simulink model "gm_hybrid_lht"  (R2019b)
settings: Solver=FixedStepDiscrete  StartTime=0.0  StopTime=inf  FixedStep=1/120e6  RelTol=1e-3
undefined symbols (not defined in the file or in its folder): bt, height, nTheta, width
libraries: hdlsllib x312, simulink x194, hdlmdlgenlib x7, dspsrcs4 x1
(part 6 of 13)

== system gm_hybrid_lht/Hybrid LHT/Hybrid LHT Accumulator/Accumulator with Switches/Accumulator_instance56 ==
  shift : Inport  OutDataTypeStr=fixdt(0, 6, 0)  PortDimensions=1  SampleTime=8.33333333333333e-09
  mode : Inport  Port=2  OutDataTypeStr=boolean  PortDimensions=1  SampleTime=8.33333333333333e-09
  address : Inport  Port=3  OutDataTypeStr=fixdt(0, 10, 0)  PortDimensions=1  SampleTime=8.33333333333333e-09
  edge : Inport  Port=4  OutDataTypeStr=boolean  PortDimensions=1  SampleTime=8.33333333333333e-09
  AND : Logic  IconShape=distinctive  AllPortsSameDT=off  OutDataTypeStr=boolean
  Add : Sum  OutDataTypeStr=fixdt(0, ceil(log2(maxRho*2)), 0)
  Bit Concat : hdlsllib/Logic and Bit Operations/Bit Concat  numInputs=2
      settings: SourceProductName=Simulink
  Bit Slice : hdlsllib/Logic and Bit Operations/Bit Slice  lidx=voteWL-1  ridx=0
  Bitwise AND : simulink/Logic and Bit Operations/Bitwise Operator  logicop=AND  UseBitMask=off  NumInputPorts=2  BitMask=bin2dec('11011001')  BitMaskRealWorld=Stored Integer
  Bitwise NOT : simulink/Logic and Bit Operations/Bitwise Operator  logicop=NOT  UseBitMask=off  BitMask=bin2dec('11011001')  BitMaskRealWorld=Stored Integer
  Bitwise OR : simulink/Logic and Bit Operations/Bitwise Operator  logicop=OR  UseBitMask=off  NumInputPorts=2  BitMask=bin2dec('11011001')  BitMaskRealWorld=Stored Integer
  Block RAM : Subsystem
  Constant : Constant  Value=0  OutDataTypeStr=fixdt(0, 36-voteWL, 0)  SampleTime=-1
  Constant1 : Constant  Value=2^(voteWL)-1  OutDataTypeStr=fixdt(0, 36, 0)  SampleTime=-1
  Delay{,1..2,4..5} (5 alike) : Delay  DelayLength=1
  Multiport Switch : MultiPortSwitch  DataPortOrder=Zero-based contiguous  Inputs=2  zeroidx=on
  Multiport Switch1 : MultiPortSwitch  DataPortOrder=Zero-based contiguous  Inputs=2  zeroidx=on
  Relational Operator : RelationalOperator  Operator===  OutDataTypeStr=boolean  RndMeth=Simplest
  Shift Arithmetic : ArithShift  BitShiftNumberSource=Input port  BitShiftNumber=8  BitShiftDirection=Left  DiagnosticForOORShift=Error
      settings: InputPortMap=u0,p1
  Shift Arithmetic1 : ArithShift  BitShiftNumberSource=Input port  BitShiftNumber=8  BitShiftDirection=Left  DiagnosticForOORShift=Error
      settings: InputPortMap=u0,p1
  Shift Arithmetic2 : ArithShift  BitShiftNumberSource=Input port  BitShiftNumber=8  BitShiftDirection=Right  DiagnosticForOORShift=Error
      settings: InputPortMap=u0,p1
  Signal Specification : SignalSpecification  OutDataTypeStr=fixdt(0, 36, 0)
  Vote : Constant  OutDataTypeStr=fixdt(0,1,0)  SampleTime=-1
  Zero : Constant  Value=0  OutDataTypeStr=fixdt(0,1,0)  SampleTime=-1
  hps : Outport
  wires:
  Block RAM/1(rd_data) -> Signal Specification/1
  Multiport Switch1/1 -> Shift Arithmetic2/1, Bitwise AND/2
  Signal Specification/1 -> Multiport Switch1/2
  Bitwise OR/1 -> Block RAM/1(wr_data), Delay5/1
  Bitwise AND/1 -> Bitwise OR/1
  Shift Arithmetic2/1 -> Bit Slice/1
  Add/1 -> Multiport Switch/3
  Multiport Switch/1 -> Bit Concat/2
  Bit Concat/1 -> Shift Arithmetic/1
  Shift Arithmetic/1 -> Bitwise OR/2
  Delay5/1 -> Multiport Switch1/3
  edge/1 -> Delay1/1
  address/1 -> Block RAM/4(rd_addr), Delay/1, Relational Operator/2
  mode/1 -> Multiport Switch/1
  shift/1 -> Delay4/1
  AND/1 -> Delay2/1
  Bit Slice/1 -> Add/2, hps/1
  Bitwise NOT/1 -> Bitwise AND/1
  Constant/1 -> Bit Concat/1
  Constant1/1 -> Shift Arithmetic1/1
  Delay/1 -> Block RAM/2(wr_addr), Relational Operator/1
  Delay1/1 -> Block RAM/3(wr_en), AND/1
  Delay2/1 -> Multiport Switch1/1
  Delay4/1 -> Shift Arithmetic2/2, Shift Arithmetic/2, Shift Arithmetic1/2
  Relational Operator/1 -> AND/2
  Shift Arithmetic1/1 -> Bitwise NOT/1
  Vote/1 -> Add/1
  Zero/1 -> Multiport Switch/2

== system gm_hybrid_lht/Hybrid LHT/Hybrid LHT Accumulator/Accumulator with Switches/Accumulator_instance57 ==
  shift : Inport  OutDataTypeStr=fixdt(0, 6, 0)  PortDimensions=1  SampleTime=8.33333333333333e-09
  mode : Inport  Port=2  OutDataTypeStr=boolean  PortDimensions=1  SampleTime=8.33333333333333e-09
  address : Inport  Port=3  OutDataTypeStr=fixdt(0, 10, 0)  PortDimensions=1  SampleTime=8.33333333333333e-09
  edge : Inport  Port=4  OutDataTypeStr=boolean  PortDimensions=1  SampleTime=8.33333333333333e-09
  AND : Logic  IconShape=distinctive  AllPortsSameDT=off  OutDataTypeStr=boolean
  Add : Sum  OutDataTypeStr=fixdt(0, ceil(log2(maxRho*2)), 0)
  Bit Concat : hdlsllib/Logic and Bit Operations/Bit Concat  numInputs=2
      settings: SourceProductName=Simulink
  Bit Slice : hdlsllib/Logic and Bit Operations/Bit Slice  lidx=voteWL-1  ridx=0
  Bitwise AND : simulink/Logic and Bit Operations/Bitwise Operator  logicop=AND  UseBitMask=off  NumInputPorts=2  BitMask=bin2dec('11011001')  BitMaskRealWorld=Stored Integer
  Bitwise NOT : simulink/Logic and Bit Operations/Bitwise Operator  logicop=NOT  UseBitMask=off  BitMask=bin2dec('11011001')  BitMaskRealWorld=Stored Integer
  Bitwise OR : simulink/Logic and Bit Operations/Bitwise Operator  logicop=OR  UseBitMask=off  NumInputPorts=2  BitMask=bin2dec('11011001')  BitMaskRealWorld=Stored Integer
  Block RAM : Subsystem
  Constant : Constant  Value=0  OutDataTypeStr=fixdt(0, 36-voteWL, 0)  SampleTime=-1
  Constant1 : Constant  Value=2^(voteWL)-1  OutDataTypeStr=fixdt(0, 36, 0)  SampleTime=-1
  Delay{,1..2,4..5} (5 alike) : Delay  DelayLength=1
  Multiport Switch : MultiPortSwitch  DataPortOrder=Zero-based contiguous  Inputs=2  zeroidx=on
  Multiport Switch1 : MultiPortSwitch  DataPortOrder=Zero-based contiguous  Inputs=2  zeroidx=on
  Relational Operator : RelationalOperator  Operator===  OutDataTypeStr=boolean  RndMeth=Simplest
  Shift Arithmetic : ArithShift  BitShiftNumberSource=Input port  BitShiftNumber=8  BitShiftDirection=Left  DiagnosticForOORShift=Error
      settings: InputPortMap=u0,p1
  Shift Arithmetic1 : ArithShift  BitShiftNumberSource=Input port  BitShiftNumber=8  BitShiftDirection=Left  DiagnosticForOORShift=Error
      settings: InputPortMap=u0,p1
  Shift Arithmetic2 : ArithShift  BitShiftNumberSource=Input port  BitShiftNumber=8  BitShiftDirection=Right  DiagnosticForOORShift=Error
      settings: InputPortMap=u0,p1
  Signal Specification : SignalSpecification  OutDataTypeStr=fixdt(0, 36, 0)
  Vote : Constant  OutDataTypeStr=fixdt(0,1,0)  SampleTime=-1
  Zero : Constant  Value=0  OutDataTypeStr=fixdt(0,1,0)  SampleTime=-1
  hps : Outport
  wires:
  Block RAM/1(rd_data) -> Signal Specification/1
  Multiport Switch1/1 -> Shift Arithmetic2/1, Bitwise AND/2
  Signal Specification/1 -> Multiport Switch1/2
  Bitwise OR/1 -> Block RAM/1(wr_data), Delay5/1
  Bitwise AND/1 -> Bitwise OR/1
  Shift Arithmetic2/1 -> Bit Slice/1
  Add/1 -> Multiport Switch/3
  Multiport Switch/1 -> Bit Concat/2
  Bit Concat/1 -> Shift Arithmetic/1
  Shift Arithmetic/1 -> Bitwise OR/2
  Delay5/1 -> Multiport Switch1/3
  edge/1 -> Delay1/1
  address/1 -> Block RAM/4(rd_addr), Delay/1, Relational Operator/2
  mode/1 -> Multiport Switch/1
  shift/1 -> Delay4/1
  AND/1 -> Delay2/1
  Bit Slice/1 -> Add/2, hps/1
  Bitwise NOT/1 -> Bitwise AND/1
  Constant/1 -> Bit Concat/1
  Constant1/1 -> Shift Arithmetic1/1
  Delay/1 -> Block RAM/2(wr_addr), Relational Operator/1
  Delay1/1 -> Block RAM/3(wr_en), AND/1
  Delay2/1 -> Multiport Switch1/1
  Delay4/1 -> Shift Arithmetic2/2, Shift Arithmetic/2, Shift Arithmetic1/2
  Relational Operator/1 -> AND/2
  Shift Arithmetic1/1 -> Bitwise NOT/1
  Vote/1 -> Add/1
  Zero/1 -> Multiport Switch/2

== system gm_hybrid_lht/Hybrid LHT/Hybrid LHT Accumulator/Accumulator with Switches/Accumulator_instance58 ==
  shift : Inport  OutDataTypeStr=fixdt(0, 6, 0)  PortDimensions=1  SampleTime=8.33333333333333e-09
  mode : Inport  Port=2  OutDataTypeStr=boolean  PortDimensions=1  SampleTime=8.33333333333333e-09
  address : Inport  Port=3  OutDataTypeStr=fixdt(0, 10, 0)  PortDimensions=1  SampleTime=8.33333333333333e-09
  edge : Inport  Port=4  OutDataTypeStr=boolean  PortDimensions=1  SampleTime=8.33333333333333e-09
  AND : Logic  IconShape=distinctive  AllPortsSameDT=off  OutDataTypeStr=boolean
  Add : Sum  OutDataTypeStr=fixdt(0, ceil(log2(maxRho*2)), 0)
  Bit Concat : hdlsllib/Logic and Bit Operations/Bit Concat  numInputs=2
      settings: SourceProductName=Simulink
  Bit Slice : hdlsllib/Logic and Bit Operations/Bit Slice  lidx=voteWL-1  ridx=0
  Bitwise AND : simulink/Logic and Bit Operations/Bitwise Operator  logicop=AND  UseBitMask=off  NumInputPorts=2  BitMask=bin2dec('11011001')  BitMaskRealWorld=Stored Integer
  Bitwise NOT : simulink/Logic and Bit Operations/Bitwise Operator  logicop=NOT  UseBitMask=off  BitMask=bin2dec('11011001')  BitMaskRealWorld=Stored Integer
  Bitwise OR : simulink/Logic and Bit Operations/Bitwise Operator  logicop=OR  UseBitMask=off  NumInputPorts=2  BitMask=bin2dec('11011001')  BitMaskRealWorld=Stored Integer
  Block RAM : Subsystem
  Constant : Constant  Value=0  OutDataTypeStr=fixdt(0, 36-voteWL, 0)  SampleTime=-1
  Constant1 : Constant  Value=2^(voteWL)-1  OutDataTypeStr=fixdt(0, 36, 0)  SampleTime=-1
  Delay{,1..2,4..5} (5 alike) : Delay  DelayLength=1
  Multiport Switch : MultiPortSwitch  DataPortOrder=Zero-based contiguous  Inputs=2  zeroidx=on
  Multiport Switch1 : MultiPortSwitch  DataPortOrder=Zero-based contiguous  Inputs=2  zeroidx=on
  Relational Operator : RelationalOperator  Operator===  OutDataTypeStr=boolean  RndMeth=Simplest
  Shift Arithmetic : ArithShift  BitShiftNumberSource=Input port  BitShiftNumber=8  BitShiftDirection=Left  DiagnosticForOORShift=Error
      settings: InputPortMap=u0,p1
  Shift Arithmetic1 : ArithShift  BitShiftNumberSource=Input port  BitShiftNumber=8  BitShiftDirection=Left  DiagnosticForOORShift=Error
      settings: InputPortMap=u0,p1
  Shift Arithmetic2 : ArithShift  BitShiftNumberSource=Input port  BitShiftNumber=8  BitShiftDirection=Right  DiagnosticForOORShift=Error
      settings: InputPortMap=u0,p1
  Signal Specification : SignalSpecification  OutDataTypeStr=fixdt(0, 36, 0)
  Vote : Constant  OutDataTypeStr=fixdt(0,1,0)  SampleTime=-1
  Zero : Constant  Value=0  OutDataTypeStr=fixdt(0,1,0)  SampleTime=-1
  hps : Outport
  wires:
  Block RAM/1(rd_data) -> Signal Specification/1
  Multiport Switch1/1 -> Shift Arithmetic2/1, Bitwise AND/2
  Signal Specification/1 -> Multiport Switch1/2
  Bitwise OR/1 -> Block RAM/1(wr_data), Delay5/1
  Bitwise AND/1 -> Bitwise OR/1
  Shift Arithmetic2/1 -> Bit Slice/1
  Add/1 -> Multiport Switch/3
  Multiport Switch/1 -> Bit Concat/2
  Bit Concat/1 -> Shift Arithmetic/1
  Shift Arithmetic/1 -> Bitwise OR/2
  Delay5/1 -> Multiport Switch1/3
  edge/1 -> Delay1/1
  address/1 -> Block RAM/4(rd_addr), Delay/1, Relational Operator/2
  mode/1 -> Multiport Switch/1
  shift/1 -> Delay4/1
  AND/1 -> Delay2/1
  Bit Slice/1 -> Add/2, hps/1
  Bitwise NOT/1 -> Bitwise AND/1
  Constant/1 -> Bit Concat/1
  Constant1/1 -> Shift Arithmetic1/1
  Delay/1 -> Block RAM/2(wr_addr), Relational Operator/1
  Delay1/1 -> Block RAM/3(wr_en), AND/1
  Delay2/1 -> Multiport Switch1/1
  Delay4/1 -> Shift Arithmetic2/2, Shift Arithmetic/2, Shift Arithmetic1/2
  Relational Operator/1 -> AND/2
  Shift Arithmetic1/1 -> Bitwise NOT/1
  Vote/1 -> Add/1
  Zero/1 -> Multiport Switch/2

== system gm_hybrid_lht/Hybrid LHT/Hybrid LHT Accumulator/Accumulator with Switches/Accumulator_instance59 ==
  shift : Inport  OutDataTypeStr=fixdt(0, 6, 0)  PortDimensions=1  SampleTime=8.33333333333333e-09
  mode : Inport  Port=2  OutDataTypeStr=boolean  PortDimensions=1  SampleTime=8.33333333333333e-09
  address : Inport  Port=3  OutDataTypeStr=fixdt(0, 10, 0)  PortDimensions=1  SampleTime=8.33333333333333e-09
  edge : Inport  Port=4  OutDataTypeStr=boolean  PortDimensions=1  SampleTime=8.33333333333333e-09
  AND : Logic  IconShape=distinctive  AllPortsSameDT=off  OutDataTypeStr=boolean
  Add : Sum  OutDataTypeStr=fixdt(0, ceil(log2(maxRho*2)), 0)
  Bit Concat : hdlsllib/Logic and Bit Operations/Bit Concat  numInputs=2
      settings: SourceProductName=Simulink
  Bit Slice : hdlsllib/Logic and Bit Operations/Bit Slice  lidx=voteWL-1  ridx=0
  Bitwise AND : simulink/Logic and Bit Operations/Bitwise Operator  logicop=AND  UseBitMask=off  NumInputPorts=2  BitMask=bin2dec('11011001')  BitMaskRealWorld=Stored Integer
  Bitwise NOT : simulink/Logic and Bit Operations/Bitwise Operator  logicop=NOT  UseBitMask=off  BitMask=bin2dec('11011001')  BitMaskRealWorld=Stored Integer
  Bitwise OR : simulink/Logic and Bit Operations/Bitwise Operator  logicop=OR  UseBitMask=off  NumInputPorts=2  BitMask=bin2dec('11011001')  BitMaskRealWorld=Stored Integer
  Block RAM : Subsystem
  Constant : Constant  Value=0  OutDataTypeStr=fixdt(0, 36-voteWL, 0)  SampleTime=-1
  Constant1 : Constant  Value=2^(voteWL)-1  OutDataTypeStr=fixdt(0, 36, 0)  SampleTime=-1
  Delay{,1..2,4..5} (5 alike) : Delay  DelayLength=1
  Multiport Switch : MultiPortSwitch  DataPortOrder=Zero-based contiguous  Inputs=2  zeroidx=on
  Multiport Switch1 : MultiPortSwitch  DataPortOrder=Zero-based contiguous  Inputs=2  zeroidx=on
  Relational Operator : RelationalOperator  Operator===  OutDataTypeStr=boolean  RndMeth=Simplest
  Shift Arithmetic : ArithShift  BitShiftNumberSource=Input port  BitShiftNumber=8  BitShiftDirection=Left  DiagnosticForOORShift=Error
      settings: InputPortMap=u0,p1
  Shift Arithmetic1 : ArithShift  BitShiftNumberSource=Input port  BitShiftNumber=8  BitShiftDirection=Left  DiagnosticForOORShift=Error
      settings: InputPortMap=u0,p1
  Shift Arithmetic2 : ArithShift  BitShiftNumberSource=Input port  BitShiftNumber=8  BitShiftDirection=Right  DiagnosticForOORShift=Error
      settings: InputPortMap=u0,p1
  Signal Specification : SignalSpecification  OutDataTypeStr=fixdt(0, 36, 0)
  Vote : Constant  OutDataTypeStr=fixdt(0,1,0)  SampleTime=-1
  Zero : Constant  Value=0  OutDataTypeStr=fixdt(0,1,0)  SampleTime=-1
  hps : Outport
  wires:
  Block RAM/1(rd_data) -> Signal Specification/1
  Multiport Switch1/1 -> Shift Arithmetic2/1, Bitwise AND/2
  Signal Specification/1 -> Multiport Switch1/2
  Bitwise OR/1 -> Block RAM/1(wr_data), Delay5/1
  Bitwise AND/1 -> Bitwise OR/1
  Shift Arithmetic2/1 -> Bit Slice/1
  Add/1 -> Multiport Switch/3
  Multiport Switch/1 -> Bit Concat/2
  Bit Concat/1 -> Shift Arithmetic/1
  Shift Arithmetic/1 -> Bitwise OR/2
  Delay5/1 -> Multiport Switch1/3
  edge/1 -> Delay1/1
  address/1 -> Block RAM/4(rd_addr), Delay/1, Relational Operator/2
  mode/1 -> Multiport Switch/1
  shift/1 -> Delay4/1
  AND/1 -> Delay2/1
  Bit Slice/1 -> Add/2, hps/1
  Bitwise NOT/1 -> Bitwise AND/1
  Constant/1 -> Bit Concat/1
  Constant1/1 -> Shift Arithmetic1/1
  Delay/1 -> Block RAM/2(wr_addr), Relational Operator/1
  Delay1/1 -> Block RAM/3(wr_en), AND/1
  Delay2/1 -> Multiport Switch1/1
  Delay4/1 -> Shift Arithmetic2/2, Shift Arithmetic/2, Shift Arithmetic1/2
  Relational Operator/1 -> AND/2
  Shift Arithmetic1/1 -> Bitwise NOT/1
  Vote/1 -> Add/1
  Zero/1 -> Multiport Switch/2

== system gm_hybrid_lht/Hybrid LHT/Hybrid LHT Accumulator/Accumulator with Switches/Accumulator_instance6 ==
  shift : Inport  OutDataTypeStr=fixdt(0, 6, 0)  PortDimensions=1  SampleTime=8.33333333333333e-09
  mode : Inport  Port=2  OutDataTypeStr=boolean  PortDimensions=1  SampleTime=8.33333333333333e-09
  address : Inport  Port=3  OutDataTypeStr=fixdt(0, 10, 0)  PortDimensions=1  SampleTime=8.33333333333333e-09
  edge : Inport  Port=4  OutDataTypeStr=boolean  PortDimensions=1  SampleTime=8.33333333333333e-09
  AND : Logic  IconShape=distinctive  AllPortsSameDT=off  OutDataTypeStr=boolean
  Add : Sum  OutDataTypeStr=fixdt(0, ceil(log2(maxRho*2)), 0)
  Bit Concat : hdlsllib/Logic and Bit Operations/Bit Concat  numInputs=2
      settings: SourceProductName=Simulink
  Bit Slice : hdlsllib/Logic and Bit Operations/Bit Slice  lidx=voteWL-1  ridx=0
  Bitwise AND : simulink/Logic and Bit Operations/Bitwise Operator  logicop=AND  UseBitMask=off  NumInputPorts=2  BitMask=bin2dec('11011001')  BitMaskRealWorld=Stored Integer
  Bitwise NOT : simulink/Logic and Bit Operations/Bitwise Operator  logicop=NOT  UseBitMask=off  BitMask=bin2dec('11011001')  BitMaskRealWorld=Stored Integer
  Bitwise OR : simulink/Logic and Bit Operations/Bitwise Operator  logicop=OR  UseBitMask=off  NumInputPorts=2  BitMask=bin2dec('11011001')  BitMaskRealWorld=Stored Integer
  Block RAM : Subsystem
  Constant : Constant  Value=0  OutDataTypeStr=fixdt(0, 36-voteWL, 0)  SampleTime=-1
  Constant1 : Constant  Value=2^(voteWL)-1  OutDataTypeStr=fixdt(0, 36, 0)  SampleTime=-1
  Delay{,1..2,4..5} (5 alike) : Delay  DelayLength=1
  Multiport Switch : MultiPortSwitch  DataPortOrder=Zero-based contiguous  Inputs=2  zeroidx=on
  Multiport Switch1 : MultiPortSwitch  DataPortOrder=Zero-based contiguous  Inputs=2  zeroidx=on
  Relational Operator : RelationalOperator  Operator===  OutDataTypeStr=boolean  RndMeth=Simplest
  Shift Arithmetic : ArithShift  BitShiftNumberSource=Input port  BitShiftNumber=8  BitShiftDirection=Left  DiagnosticForOORShift=Error
      settings: InputPortMap=u0,p1
  Shift Arithmetic1 : ArithShift  BitShiftNumberSource=Input port  BitShiftNumber=8  BitShiftDirection=Left  DiagnosticForOORShift=Error
      settings: InputPortMap=u0,p1
  Shift Arithmetic2 : ArithShift  BitShiftNumberSource=Input port  BitShiftNumber=8  BitShiftDirection=Right  DiagnosticForOORShift=Error
      settings: InputPortMap=u0,p1
  Signal Specification : SignalSpecification  OutDataTypeStr=fixdt(0, 36, 0)
  Vote : Constant  OutDataTypeStr=fixdt(0,1,0)  SampleTime=-1
  Zero : Constant  Value=0  OutDataTypeStr=fixdt(0,1,0)  SampleTime=-1
  hps : Outport
  wires:
  Block RAM/1(rd_data) -> Signal Specification/1
  Multiport Switch1/1 -> Shift Arithmetic2/1, Bitwise AND/2
  Signal Specification/1 -> Multiport Switch1/2
  Bitwise OR/1 -> Block RAM/1(wr_data), Delay5/1
  Bitwise AND/1 -> Bitwise OR/1
  Shift Arithmetic2/1 -> Bit Slice/1
  Add/1 -> Multiport Switch/3
  Multiport Switch/1 -> Bit Concat/2
  Bit Concat/1 -> Shift Arithmetic/1
  Shift Arithmetic/1 -> Bitwise OR/2
  Delay5/1 -> Multiport Switch1/3
  edge/1 -> Delay1/1
  address/1 -> Block RAM/4(rd_addr), Delay/1, Relational Operator/2
  mode/1 -> Multiport Switch/1
  shift/1 -> Delay4/1
  AND/1 -> Delay2/1
  Bit Slice/1 -> Add/2, hps/1
  Bitwise NOT/1 -> Bitwise AND/1
  Constant/1 -> Bit Concat/1
  Constant1/1 -> Shift Arithmetic1/1
  Delay/1 -> Block RAM/2(wr_addr), Relational Operator/1
  Delay1/1 -> Block RAM/3(wr_en), AND/1
  Delay2/1 -> Multiport Switch1/1
  Delay4/1 -> Shift Arithmetic2/2, Shift Arithmetic/2, Shift Arithmetic1/2
  Relational Operator/1 -> AND/2
  Shift Arithmetic1/1 -> Bitwise NOT/1
  Vote/1 -> Add/1
  Zero/1 -> Multiport Switch/2

== system gm_hybrid_lht/Hybrid LHT/Hybrid LHT Accumulator/Accumulator with Switches/Accumulator_instance60 ==
  shift : Inport  OutDataTypeStr=fixdt(0, 6, 0)  PortDimensions=1  SampleTime=8.33333333333333e-09
  mode : Inport  Port=2  OutDataTypeStr=boolean  PortDimensions=1  SampleTime=8.33333333333333e-09
  address : Inport  Port=3  OutDataTypeStr=fixdt(0, 10, 0)  PortDimensions=1  SampleTime=8.33333333333333e-09
  edge : Inport  Port=4  OutDataTypeStr=boolean  PortDimensions=1  SampleTime=8.33333333333333e-09
  AND : Logic  IconShape=distinctive  AllPortsSameDT=off  OutDataTypeStr=boolean
  Add : Sum  OutDataTypeStr=fixdt(0, ceil(log2(maxRho*2)), 0)
  Bit Concat : hdlsllib/Logic and Bit Operations/Bit Concat  numInputs=2
      settings: SourceProductName=Simulink
  Bit Slice : hdlsllib/Logic and Bit Operations/Bit Slice  lidx=voteWL-1  ridx=0
  Bitwise AND : simulink/Logic and Bit Operations/Bitwise Operator  logicop=AND  UseBitMask=off  NumInputPorts=2  BitMask=bin2dec('11011001')  BitMaskRealWorld=Stored Integer
  Bitwise NOT : simulink/Logic and Bit Operations/Bitwise Operator  logicop=NOT  UseBitMask=off  BitMask=bin2dec('11011001')  BitMaskRealWorld=Stored Integer
  Bitwise OR : simulink/Logic and Bit Operations/Bitwise Operator  logicop=OR  UseBitMask=off  NumInputPorts=2  BitMask=bin2dec('11011001')  BitMaskRealWorld=Stored Integer
  Block RAM : Subsystem
  Constant : Constant  Value=0  OutDataTypeStr=fixdt(0, 36-voteWL, 0)  SampleTime=-1
  Constant1 : Constant  Value=2^(voteWL)-1  OutDataTypeStr=fixdt(0, 36, 0)  SampleTime=-1
  Delay{,1..2,4..5} (5 alike) : Delay  DelayLength=1
  Multiport Switch : MultiPortSwitch  DataPortOrder=Zero-based contiguous  Inputs=2  zeroidx=on
  Multiport Switch1 : MultiPortSwitch  DataPortOrder=Zero-based contiguous  Inputs=2  zeroidx=on
  Relational Operator : RelationalOperator  Operator===  OutDataTypeStr=boolean  RndMeth=Simplest
  Shift Arithmetic : ArithShift  BitShiftNumberSource=Input port  BitShiftNumber=8  BitShiftDirection=Left  DiagnosticForOORShift=Error
      settings: InputPortMap=u0,p1
  Shift Arithmetic1 : ArithShift  BitShiftNumberSource=Input port  BitShiftNumber=8  BitShiftDirection=Left  DiagnosticForOORShift=Error
      settings: InputPortMap=u0,p1
  Shift Arithmetic2 : ArithShift  BitShiftNumberSource=Input port  BitShiftNumber=8  BitShiftDirection=Right  DiagnosticForOORShift=Error
      settings: InputPortMap=u0,p1
  Signal Specification : SignalSpecification  OutDataTypeStr=fixdt(0, 36, 0)
  Vote : Constant  OutDataTypeStr=fixdt(0,1,0)  SampleTime=-1
  Zero : Constant  Value=0  OutDataTypeStr=fixdt(0,1,0)  SampleTime=-1
  hps : Outport
  wires:
  Block RAM/1(rd_data) -> Signal Specification/1
  Multiport Switch1/1 -> Shift Arithmetic2/1, Bitwise AND/2
  Signal Specification/1 -> Multiport Switch1/2
  Bitwise OR/1 -> Block RAM/1(wr_data), Delay5/1
  Bitwise AND/1 -> Bitwise OR/1
  Shift Arithmetic2/1 -> Bit Slice/1
  Add/1 -> Multiport Switch/3
  Multiport Switch/1 -> Bit Concat/2
  Bit Concat/1 -> Shift Arithmetic/1
  Shift Arithmetic/1 -> Bitwise OR/2
  Delay5/1 -> Multiport Switch1/3
  edge/1 -> Delay1/1
  address/1 -> Block RAM/4(rd_addr), Delay/1, Relational Operator/2
  mode/1 -> Multiport Switch/1
  shift/1 -> Delay4/1
  AND/1 -> Delay2/1
  Bit Slice/1 -> Add/2, hps/1
  Bitwise NOT/1 -> Bitwise AND/1
  Constant/1 -> Bit Concat/1
  Constant1/1 -> Shift Arithmetic1/1
  Delay/1 -> Block RAM/2(wr_addr), Relational Operator/1
  Delay1/1 -> Block RAM/3(wr_en), AND/1
  Delay2/1 -> Multiport Switch1/1
  Delay4/1 -> Shift Arithmetic2/2, Shift Arithmetic/2, Shift Arithmetic1/2
  Relational Operator/1 -> AND/2
  Shift Arithmetic1/1 -> Bitwise NOT/1
  Vote/1 -> Add/1
  Zero/1 -> Multiport Switch/2

== system gm_hybrid_lht/Hybrid LHT/Hybrid LHT Accumulator/Accumulator with Switches/Accumulator_instance7 ==
  shift : Inport  OutDataTypeStr=fixdt(0, 6, 0)  PortDimensions=1  SampleTime=8.33333333333333e-09
  mode : Inport  Port=2  OutDataTypeStr=boolean  PortDimensions=1  SampleTime=8.33333333333333e-09
  address : Inport  Port=3  OutDataTypeStr=fixdt(0, 10, 0)  PortDimensions=1  SampleTime=8.33333333333333e-09
  edge : Inport  Port=4  OutDataTypeStr=boolean  PortDimensions=1  SampleTime=8.33333333333333e-09
  AND : Logic  IconShape=distinctive  AllPortsSameDT=off  OutDataTypeStr=boolean
  Add : Sum  OutDataTypeStr=fixdt(0, ceil(log2(maxRho*2)), 0)
  Bit Concat : hdlsllib/Logic and Bit Operations/Bit Concat  numInputs=2
      settings: SourceProductName=Simulink
  Bit Slice : hdlsllib/Logic and Bit Operations/Bit Slice  lidx=voteWL-1  ridx=0
  Bitwise AND : simulink/Logic and Bit Operations/Bitwise Operator  logicop=AND  UseBitMask=off  NumInputPorts=2  BitMask=bin2dec('11011001')  BitMaskRealWorld=Stored Integer
  Bitwise NOT : simulink/Logic and Bit Operations/Bitwise Operator  logicop=NOT  UseBitMask=off  BitMask=bin2dec('11011001')  BitMaskRealWorld=Stored Integer
  Bitwise OR : simulink/Logic and Bit Operations/Bitwise Operator  logicop=OR  UseBitMask=off  NumInputPorts=2  BitMask=bin2dec('11011001')  BitMaskRealWorld=Stored Integer
  Block RAM : Subsystem
  Constant : Constant  Value=0  OutDataTypeStr=fixdt(0, 36-voteWL, 0)  SampleTime=-1
  Constant1 : Constant  Value=2^(voteWL)-1  OutDataTypeStr=fixdt(0, 36, 0)  SampleTime=-1
  Delay{,1..2,4..5} (5 alike) : Delay  DelayLength=1
  Multiport Switch : MultiPortSwitch  DataPortOrder=Zero-based contiguous  Inputs=2  zeroidx=on
  Multiport Switch1 : MultiPortSwitch  DataPortOrder=Zero-based contiguous  Inputs=2  zeroidx=on
  Relational Operator : RelationalOperator  Operator===  OutDataTypeStr=boolean  RndMeth=Simplest
  Shift Arithmetic : ArithShift  BitShiftNumberSource=Input port  BitShiftNumber=8  BitShiftDirection=Left  DiagnosticForOORShift=Error
      settings: InputPortMap=u0,p1
  Shift Arithmetic1 : ArithShift  BitShiftNumberSource=Input port  BitShiftNumber=8  BitShiftDirection=Left  DiagnosticForOORShift=Error
      settings: InputPortMap=u0,p1
  Shift Arithmetic2 : ArithShift  BitShiftNumberSource=Input port  BitShiftNumber=8  BitShiftDirection=Right  DiagnosticForOORShift=Error
      settings: InputPortMap=u0,p1
  Signal Specification : SignalSpecification  OutDataTypeStr=fixdt(0, 36, 0)
  Vote : Constant  OutDataTypeStr=fixdt(0,1,0)  SampleTime=-1
  Zero : Constant  Value=0  OutDataTypeStr=fixdt(0,1,0)  SampleTime=-1
  hps : Outport
  wires:
  Block RAM/1(rd_data) -> Signal Specification/1
  Multiport Switch1/1 -> Shift Arithmetic2/1, Bitwise AND/2
  Signal Specification/1 -> Multiport Switch1/2
  Bitwise OR/1 -> Block RAM/1(wr_data), Delay5/1
  Bitwise AND/1 -> Bitwise OR/1
  Shift Arithmetic2/1 -> Bit Slice/1
  Add/1 -> Multiport Switch/3
  Multiport Switch/1 -> Bit Concat/2
  Bit Concat/1 -> Shift Arithmetic/1
  Shift Arithmetic/1 -> Bitwise OR/2
  Delay5/1 -> Multiport Switch1/3
  edge/1 -> Delay1/1
  address/1 -> Block RAM/4(rd_addr), Delay/1, Relational Operator/2
  mode/1 -> Multiport Switch/1
  shift/1 -> Delay4/1
  AND/1 -> Delay2/1
  Bit Slice/1 -> Add/2, hps/1
  Bitwise NOT/1 -> Bitwise AND/1
  Constant/1 -> Bit Concat/1
  Constant1/1 -> Shift Arithmetic1/1
  Delay/1 -> Block RAM/2(wr_addr), Relational Operator/1
  Delay1/1 -> Block RAM/3(wr_en), AND/1
  Delay2/1 -> Multiport Switch1/1
  Delay4/1 -> Shift Arithmetic2/2, Shift Arithmetic/2, Shift Arithmetic1/2
  Relational Operator/1 -> AND/2
  Shift Arithmetic1/1 -> Bitwise NOT/1
  Vote/1 -> Add/1
  Zero/1 -> Multiport Switch/2

== system gm_hybrid_lht/Hybrid LHT/Hybrid LHT Accumulator/Accumulator with Switches/Accumulator_instance8 ==
  shift : Inport  OutDataTypeStr=fixdt(0, 6, 0)  PortDimensions=1  SampleTime=8.33333333333333e-09
  mode : Inport  Port=2  OutDataTypeStr=boolean  PortDimensions=1  SampleTime=8.33333333333333e-09
  address : Inport  Port=3  OutDataTypeStr=fixdt(0, 10, 0)  PortDimensions=1  SampleTime=8.33333333333333e-09
  edge : Inport  Port=4  OutDataTypeStr=boolean  PortDimensions=1  SampleTime=8.33333333333333e-09
  AND : Logic  IconShape=distinctive  AllPortsSameDT=off  OutDataTypeStr=boolean
  Add : Sum  OutDataTypeStr=fixdt(0, ceil(log2(maxRho*2)), 0)
  Bit Concat : hdlsllib/Logic and Bit Operations/Bit Concat  numInputs=2
      settings: SourceProductName=Simulink
  Bit Slice : hdlsllib/Logic and Bit Operations/Bit Slice  lidx=voteWL-1  ridx=0
  Bitwise AND : simulink/Logic and Bit Operations/Bitwise Operator  logicop=AND  UseBitMask=off  NumInputPorts=2  BitMask=bin2dec('11011001')  BitMaskRealWorld=Stored Integer
  Bitwise NOT : simulink/Logic and Bit Operations/Bitwise Operator  logicop=NOT  UseBitMask=off  BitMask=bin2dec('11011001')  BitMaskRealWorld=Stored Integer
  Bitwise OR : simulink/Logic and Bit Operations/Bitwise Operator  logicop=OR  UseBitMask=off  NumInputPorts=2  BitMask=bin2dec('11011001')  BitMaskRealWorld=Stored Integer
  Block RAM : Subsystem
  Constant : Constant  Value=0  OutDataTypeStr=fixdt(0, 36-voteWL, 0)  SampleTime=-1
  Constant1 : Constant  Value=2^(voteWL)-1  OutDataTypeStr=fixdt(0, 36, 0)  SampleTime=-1
  Delay{,1..2,4..5} (5 alike) : Delay  DelayLength=1
  Multiport Switch : MultiPortSwitch  DataPortOrder=Zero-based contiguous  Inputs=2  zeroidx=on
  Multiport Switch1 : MultiPortSwitch  DataPortOrder=Zero-based contiguous  Inputs=2  zeroidx=on
  Relational Operator : RelationalOperator  Operator===  OutDataTypeStr=boolean  RndMeth=Simplest
  Shift Arithmetic : ArithShift  BitShiftNumberSource=Input port  BitShiftNumber=8  BitShiftDirection=Left  DiagnosticForOORShift=Error
      settings: InputPortMap=u0,p1
  Shift Arithmetic1 : ArithShift  BitShiftNumberSource=Input port  BitShiftNumber=8  BitShiftDirection=Left  DiagnosticForOORShift=Error
      settings: InputPortMap=u0,p1
  Shift Arithmetic2 : ArithShift  BitShiftNumberSource=Input port  BitShiftNumber=8  BitShiftDirection=Right  DiagnosticForOORShift=Error
      settings: InputPortMap=u0,p1
  Signal Specification : SignalSpecification  OutDataTypeStr=fixdt(0, 36, 0)
  Vote : Constant  OutDataTypeStr=fixdt(0,1,0)  SampleTime=-1
  Zero : Constant  Value=0  OutDataTypeStr=fixdt(0,1,0)  SampleTime=-1
  hps : Outport
  wires:
  Block RAM/1(rd_data) -> Signal Specification/1
  Multiport Switch1/1 -> Shift Arithmetic2/1, Bitwise AND/2
  Signal Specification/1 -> Multiport Switch1/2
  Bitwise OR/1 -> Block RAM/1(wr_data), Delay5/1
  Bitwise AND/1 -> Bitwise OR/1
  Shift Arithmetic2/1 -> Bit Slice/1
  Add/1 -> Multiport Switch/3
  Multiport Switch/1 -> Bit Concat/2
  Bit Concat/1 -> Shift Arithmetic/1
  Shift Arithmetic/1 -> Bitwise OR/2
  Delay5/1 -> Multiport Switch1/3
  edge/1 -> Delay1/1
  address/1 -> Block RAM/4(rd_addr), Delay/1, Relational Operator/2
  mode/1 -> Multiport Switch/1
  shift/1 -> Delay4/1
  AND/1 -> Delay2/1
  Bit Slice/1 -> Add/2, hps/1
  Bitwise NOT/1 -> Bitwise AND/1
  Constant/1 -> Bit Concat/1
  Constant1/1 -> Shift Arithmetic1/1
  Delay/1 -> Block RAM/2(wr_addr), Relational Operator/1
  Delay1/1 -> Block RAM/3(wr_en), AND/1
  Delay2/1 -> Multiport Switch1/1
  Delay4/1 -> Shift Arithmetic2/2, Shift Arithmetic/2, Shift Arithmetic1/2
  Relational Operator/1 -> AND/2
  Shift Arithmetic1/1 -> Bitwise NOT/1
  Vote/1 -> Add/1
  Zero/1 -> Multiport Switch/2

== system gm_hybrid_lht/Hybrid LHT/Hybrid LHT Accumulator/Accumulator with Switches/Accumulator_instance9 ==
  shift : Inport  OutDataTypeStr=fixdt(0, 6, 0)  PortDimensions=1  SampleTime=8.33333333333333e-09
  mode : Inport  Port=2  OutDataTypeStr=boolean  PortDimensions=1  SampleTime=8.33333333333333e-09
  address : Inport  Port=3  OutDataTypeStr=fixdt(0, 10, 0)  PortDimensions=1  SampleTime=8.33333333333333e-09
  edge : Inport  Port=4  OutDataTypeStr=boolean  PortDimensions=1  SampleTime=8.33333333333333e-09
  AND : Logic  IconShape=distinctive  AllPortsSameDT=off  OutDataTypeStr=boolean
  Add : Sum  OutDataTypeStr=fixdt(0, ceil(log2(maxRho*2)), 0)
  Bit Concat : hdlsllib/Logic and Bit Operations/Bit Concat  numInputs=2
      settings: SourceProductName=Simulink
  Bit Slice : hdlsllib/Logic and Bit Operations/Bit Slice  lidx=voteWL-1  ridx=0
  Bitwise AND : simulink/Logic and Bit Operations/Bitwise Operator  logicop=AND  UseBitMask=off  NumInputPorts=2  BitMask=bin2dec('11011001')  BitMaskRealWorld=Stored Integer
  Bitwise NOT : simulink/Logic and Bit Operations/Bitwise Operator  logicop=NOT  UseBitMask=off  BitMask=bin2dec('11011001')  BitMaskRealWorld=Stored Integer
  Bitwise OR : simulink/Logic and Bit Operations/Bitwise Operator  logicop=OR  UseBitMask=off  NumInputPorts=2  BitMask=bin2dec('11011001')  BitMaskRealWorld=Stored Integer
  Block RAM : Subsystem
  Constant : Constant  Value=0  OutDataTypeStr=fixdt(0, 36-voteWL, 0)  SampleTime=-1
  Constant1 : Constant  Value=2^(voteWL)-1  OutDataTypeStr=fixdt(0, 36, 0)  SampleTime=-1
  Delay{,1..2,4..5} (5 alike) : Delay  DelayLength=1
  Multiport Switch : MultiPortSwitch  DataPortOrder=Zero-based contiguous  Inputs=2  zeroidx=on
  Multiport Switch1 : MultiPortSwitch  DataPortOrder=Zero-based contiguous  Inputs=2  zeroidx=on
  Relational Operator : RelationalOperator  Operator===  OutDataTypeStr=boolean  RndMeth=Simplest
  Shift Arithmetic : ArithShift  BitShiftNumberSource=Input port  BitShiftNumber=8  BitShiftDirection=Left  DiagnosticForOORShift=Error
      settings: InputPortMap=u0,p1
  Shift Arithmetic1 : ArithShift  BitShiftNumberSource=Input port  BitShiftNumber=8  BitShiftDirection=Left  DiagnosticForOORShift=Error
      settings: InputPortMap=u0,p1
  Shift Arithmetic2 : ArithShift  BitShiftNumberSource=Input port  BitShiftNumber=8  BitShiftDirection=Right  DiagnosticForOORShift=Error
      settings: InputPortMap=u0,p1
  Signal Specification : SignalSpecification  OutDataTypeStr=fixdt(0, 36, 0)
  Vote : Constant  OutDataTypeStr=fixdt(0,1,0)  SampleTime=-1
  Zero : Constant  Value=0  OutDataTypeStr=fixdt(0,1,0)  SampleTime=-1
  hps : Outport
  wires:
  Block RAM/1(rd_data) -> Signal Specification/1
  Multiport Switch1/1 -> Shift Arithmetic2/1, Bitwise AND/2
  Signal Specification/1 -> Multiport Switch1/2
  Bitwise OR/1 -> Block RAM/1(wr_data), Delay5/1
  Bitwise AND/1 -> Bitwise OR/1
  Shift Arithmetic2/1 -> Bit Slice/1
  Add/1 -> Multiport Switch/3
  Multiport Switch/1 -> Bit Concat/2
  Bit Concat/1 -> Shift Arithmetic/1
  Shift Arithmetic/1 -> Bitwise OR/2
  Delay5/1 -> Multiport Switch1/3
  edge/1 -> Delay1/1
  address/1 -> Block RAM/4(rd_addr), Delay/1, Relational Operator/2
  mode/1 -> Multiport Switch/1
  shift/1 -> Delay4/1
  AND/1 -> Delay2/1
  Bit Slice/1 -> Add/2, hps/1
  Bitwise NOT/1 -> Bitwise AND/1
  Constant/1 -> Bit Concat/1
  Constant1/1 -> Shift Arithmetic1/1
  Delay/1 -> Block RAM/2(wr_addr), Relational Operator/1
  Delay1/1 -> Block RAM/3(wr_en), AND/1
  Delay2/1 -> Multiport Switch1/1
  Delay4/1 -> Shift Arithmetic2/2, Shift Arithmetic/2, Shift Arithmetic1/2
  Relational Operator/1 -> AND/2
  Shift Arithmetic1/1 -> Bitwise NOT/1
  Vote/1 -> Add/1
  Zero/1 -> Multiport Switch/2

== system gm_hybrid_lht/Hybrid LHT/Hybrid LHT Kernel/Extract Active Votes/GetShift ==
  Theta : Inport  OutDataTypeStr=uint8  PortDimensions=1  SampleTime=8.33333333333333e-09
  Add : Sum  Inputs=+  OutDataTypeStr=fixdt(0, ceil(log2(L+1)), 0)
  Constant : Constant  Value=U  VectorParams1D=off  OutDataTypeStr=fixdt(0,ceil(log2(max(U)+1)),0)  SampleTime=-1
  Relational Operator : RelationalOperator  OutDataTypeStr=boolean  RndMeth=Nearest
  Shift : Outport  VectorParamsAs1DForOutWhenUnconnected=off
  wires:
  Add/1 -> Shift/1
  Constant/1 -> Relational Operator/2
  Relational Operator/1 -> Add/1
  Theta/1 -> Relational Operator/1

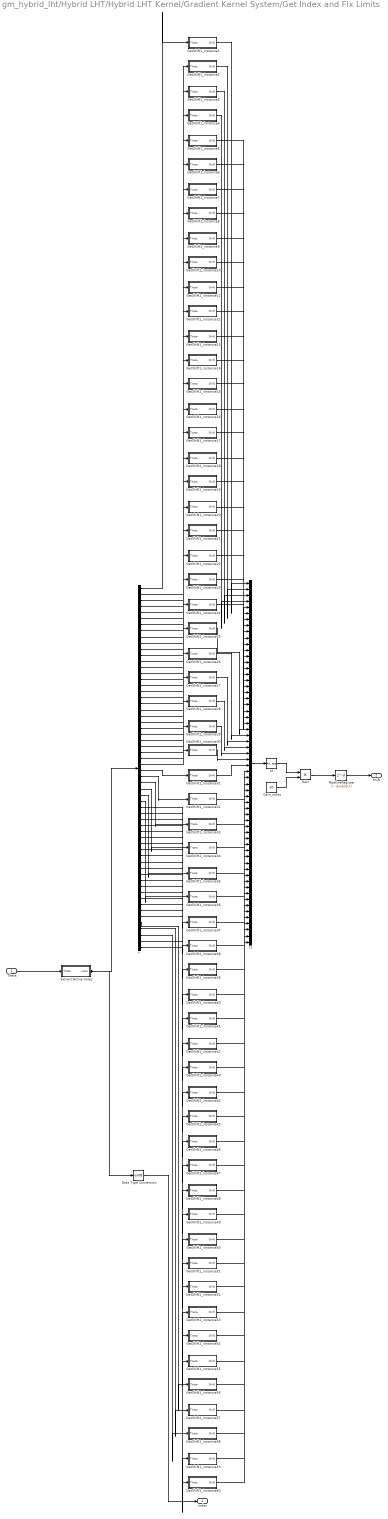
== system gm_hybrid_lht/Hybrid LHT/Hybrid LHT Kernel/Gradient Kernel System/Get Index and Fix Limits ==
  Theta : Inport  OutDataTypeStr=uint8  PortDimensions=1  SampleTime=8.33333333333333e-09
  Data Type Conversion : DataTypeConversion  OutDataTypeStr=uint8  SampleTime=8.33333333333333e-09
  Extract Active Votes : Subsystem
  Gain : Product  Inputs=**  OutDataTypeStr=fixdt(0, 6, 0)  SampleTime=8.33333333333333e-09
  Gain_const : Constant  Value=10  OutDataTypeStr=fixdt(0, 6, 0)  SampleTime=-1
  GetShift1_instance1 : Subsystem
  GetShift1_instance10 : Subsystem
  GetShift1_instance11 : Subsystem
  GetShift1_instance12 : Subsystem
  GetShift1_instance13 : Subsystem
  GetShift1_instance14 : Subsystem
  GetShift1_instance15 : Subsystem
  GetShift1_instance16 : Subsystem
  GetShift1_instance17 : Subsystem
  GetShift1_instance18 : Subsystem
  GetShift1_instance19 : Subsystem
  GetShift1_instance2 : Subsystem
  GetShift1_instance20 : Subsystem
  GetShift1_instance21 : Subsystem
  GetShift1_instance22 : Subsystem
  GetShift1_instance23 : Subsystem
  GetShift1_instance24 : Subsystem
  GetShift1_instance25 : Subsystem
  GetShift1_instance26 : Subsystem
  GetShift1_instance27 : Subsystem
  GetShift1_instance28 : Subsystem
  GetShift1_instance29 : Subsystem
  GetShift1_instance3 : Subsystem
  GetShift1_instance30 : Subsystem
  GetShift1_instance31 : Subsystem
  GetShift1_instance32 : Subsystem
  GetShift1_instance33 : Subsystem
  GetShift1_instance34 : Subsystem
  GetShift1_instance35 : Subsystem
  GetShift1_instance36 : Subsystem
  GetShift1_instance37 : Subsystem
  GetShift1_instance38 : Subsystem
  GetShift1_instance39 : Subsystem
  GetShift1_instance4 : Subsystem
  GetShift1_instance40 : Subsystem
  GetShift1_instance41 : Subsystem
  GetShift1_instance42 : Subsystem
  GetShift1_instance43 : Subsystem
  GetShift1_instance44 : Subsystem
  GetShift1_instance45 : Subsystem
  GetShift1_instance46 : Subsystem
  GetShift1_instance47 : Subsystem
  GetShift1_instance48 : Subsystem
  GetShift1_instance49 : Subsystem
  GetShift1_instance5 : Subsystem
  GetShift1_instance50 : Subsystem
  GetShift1_instance51 : Subsystem
  GetShift1_instance52 : Subsystem
  GetShift1_instance53 : Subsystem
  GetShift1_instance54 : Subsystem
  GetShift1_instance55 : Subsystem
  GetShift1_instance56 : Subsystem
  GetShift1_instance57 : Subsystem
  GetShift1_instance58 : Subsystem
  GetShift1_instance59 : Subsystem
  GetShift1_instance6 : Subsystem
  GetShift1_instance60 : Subsystem
  GetShift1_instance7 : Subsystem
  GetShift1_instance8 : Subsystem
  GetShift1_instance9 : Subsystem
  PipelineRegister : Delay  DelayLength=double(1)  InitialCondition=0  SampleTime=8.33333333333333e-09
  t : Demux  Outputs=60
  t1 : Concatenate  NumInputs=60
  t2 : Reshape  OutputDimensionality=Row vector (2-D)
  Index : Outport  VectorParamsAs1DForOutWhenUnconnected=off
  Shift : Outport  Port=2  VectorParamsAs1DForOutWhenUnconnected=off
  wires:
  Data Type Conversion/1 -> Index/1
  Extract Active Votes/1(Index) -> Data Type Conversion/1, t/1
  PipelineRegister/1 -> Shift/1
  t2/1 -> Gain/1
  t/1 -> GetShift1_instance1/1(Theta)
  t/2 -> GetShift1_instance2/1(Theta)
  t/3 -> GetShift1_instance3/1(Theta)
  t/4 -> GetShift1_instance4/1(Theta)
  t/5 -> GetShift1_instance5/1(Theta)
  t/6 -> GetShift1_instance6/1(Theta)
  t/7 -> GetShift1_instance7/1(Theta)
  t/8 -> GetShift1_instance8/1(Theta)
  t/9 -> GetShift1_instance9/1(Theta)
  t/10 -> GetShift1_instance10/1(Theta)
  t/11 -> GetShift1_instance11/1(Theta)
  t/12 -> GetShift1_instance12/1(Theta)
  t/13 -> GetShift1_instance13/1(Theta)
  t/14 -> GetShift1_instance14/1(Theta)
  t/15 -> GetShift1_instance15/1(Theta)
  t/16 -> GetShift1_instance16/1(Theta)
  t/17 -> GetShift1_instance17/1(Theta)
  t/18 -> GetShift1_instance18/1(Theta)
  t/19 -> GetShift1_instance19/1(Theta)
  t/20 -> GetShift1_instance20/1(Theta)
  t/21 -> GetShift1_instance21/1(Theta)
  t/22 -> GetShift1_instance22/1(Theta)
  t/23 -> GetShift1_instance23/1(Theta)
  t/24 -> GetShift1_instance24/1(Theta)
  t/25 -> GetShift1_instance25/1(Theta)
  t/26 -> GetShift1_instance26/1(Theta)
  t/27 -> GetShift1_instance27/1(Theta)
  t/28 -> GetShift1_instance28/1(Theta)
  t/29 -> GetShift1_instance29/1(Theta)
  t/30 -> GetShift1_instance30/1(Theta)
  t/31 -> GetShift1_instance31/1(Theta)
  t/32 -> GetShift1_instance32/1(Theta)
  t/33 -> GetShift1_instance33/1(Theta)
  t/34 -> GetShift1_instance34/1(Theta)
  t/35 -> GetShift1_instance35/1(Theta)
  t/36 -> GetShift1_instance36/1(Theta)
  t/37 -> GetShift1_instance37/1(Theta)
  t/38 -> GetShift1_instance38/1(Theta)
  t/39 -> GetShift1_instance39/1(Theta)
  t/40 -> GetShift1_instance40/1(Theta)
  t/41 -> GetShift1_instance41/1(Theta)
  t/42 -> GetShift1_instance42/1(Theta)
  t/43 -> GetShift1_instance43/1(Theta)
  t/44 -> GetShift1_instance44/1(Theta)
  t/45 -> GetShift1_instance45/1(Theta)
  t/46 -> GetShift1_instance46/1(Theta)
  t/47 -> GetShift1_instance47/1(Theta)
  t/48 -> GetShift1_instance48/1(Theta)
  t/49 -> GetShift1_instance49/1(Theta)
  t/50 -> GetShift1_instance50/1(Theta)
  t/51 -> GetShift1_instance51/1(Theta)
  t/52 -> GetShift1_instance52/1(Theta)
  t/53 -> GetShift1_instance53/1(Theta)
  t/54 -> GetShift1_instance54/1(Theta)
  t/55 -> GetShift1_instance55/1(Theta)
  t/56 -> GetShift1_instance56/1(Theta)
  t/57 -> GetShift1_instance57/1(Theta)
  t/58 -> GetShift1_instance58/1(Theta)
  t/59 -> GetShift1_instance59/1(Theta)
  t/60 -> GetShift1_instance60/1(Theta)
  t1/1 -> t2/1
  GetShift1_instance1/1(Shift) -> t1/1
  GetShift1_instance2/1(Shift) -> t1/2
  GetShift1_instance3/1(Shift) -> t1/3
  GetShift1_instance4/1(Shift) -> t1/4
  GetShift1_instance5/1(Shift) -> t1/5
  GetShift1_instance6/1(Shift) -> t1/6
  GetShift1_instance7/1(Shift) -> t1/7
  GetShift1_instance8/1(Shift) -> t1/8
  GetShift1_instance9/1(Shift) -> t1/9
  GetShift1_instance10/1(Shift) -> t1/10
  GetShift1_instance11/1(Shift) -> t1/11
  GetShift1_instance12/1(Shift) -> t1/12
  GetShift1_instance13/1(Shift) -> t1/13
  GetShift1_instance14/1(Shift) -> t1/14
  GetShift1_instance15/1(Shift) -> t1/15
  GetShift1_instance16/1(Shift) -> t1/16
  GetShift1_instance17/1(Shift) -> t1/17
  GetShift1_instance18/1(Shift) -> t1/18
  GetShift1_instance19/1(Shift) -> t1/19
  GetShift1_instance20/1(Shift) -> t1/20
  GetShift1_instance21/1(Shift) -> t1/21
  GetShift1_instance22/1(Shift) -> t1/22
  GetShift1_instance23/1(Shift) -> t1/23
  GetShift1_instance24/1(Shift) -> t1/24
  GetShift1_instance25/1(Shift) -> t1/25
  GetShift1_instance26/1(Shift) -> t1/26
  GetShift1_instance27/1(Shift) -> t1/27
  GetShift1_instance28/1(Shift) -> t1/28
  GetShift1_instance29/1(Shift) -> t1/29
  GetShift1_instance30/1(Shift) -> t1/30
  GetShift1_instance31/1(Shift) -> t1/31
  GetShift1_instance32/1(Shift) -> t1/32
  GetShift1_instance33/1(Shift) -> t1/33
  GetShift1_instance34/1(Shift) -> t1/34
  GetShift1_instance35/1(Shift) -> t1/35
  GetShift1_instance36/1(Shift) -> t1/36
  GetShift1_instance37/1(Shift) -> t1/37
  GetShift1_instance38/1(Shift) -> t1/38
  GetShift1_instance39/1(Shift) -> t1/39
  GetShift1_instance40/1(Shift) -> t1/40
  GetShift1_instance41/1(Shift) -> t1/41
  GetShift1_instance42/1(Shift) -> t1/42
  GetShift1_instance43/1(Shift) -> t1/43
  GetShift1_instance44/1(Shift) -> t1/44
  GetShift1_instance45/1(Shift) -> t1/45
  GetShift1_instance46/1(Shift) -> t1/46
  GetShift1_instance47/1(Shift) -> t1/47
  GetShift1_instance48/1(Shift) -> t1/48
  GetShift1_instance49/1(Shift) -> t1/49
  GetShift1_instance50/1(Shift) -> t1/50
  GetShift1_instance51/1(Shift) -> t1/51
  GetShift1_instance52/1(Shift) -> t1/52
  GetShift1_instance53/1(Shift) -> t1/53
  GetShift1_instance54/1(Shift) -> t1/54
  GetShift1_instance55/1(Shift) -> t1/55
  GetShift1_instance56/1(Shift) -> t1/56
  GetShift1_instance57/1(Shift) -> t1/57
  GetShift1_instance58/1(Shift) -> t1/58
  GetShift1_instance59/1(Shift) -> t1/59
  GetShift1_instance60/1(Shift) -> t1/60
  Gain_const/1 -> Gain/2
  Theta/1 -> Extract Active Votes/1(Theta)
  Gain/1 -> PipelineRegister/1

== system gm_hybrid_lht/Hybrid LHT/Hybrid LHT Kernel/Gradient Kernel System/Hough Kernel ==
  Edge : Inport  OutDataTypeStr=fixdt(0, 1, 0)  PortDimensions=1  SampleTime=8.33333333333333e-09
  X : Inport  Port=2  OutDataTypeStr=fixdt(1, 9, 0)  PortDimensions=1  SampleTime=8.33333333333333e-09
  Y : Inport  Port=3  OutDataTypeStr=fixdt(1, 9, 0)  PortDimensions=1  SampleTime=8.33333333333333e-09
  Index : Inport  Port=4  OutDataTypeStr=uint8  PortDimensions=[1 60]  SampleTime=8.33333333333333e-09
  Add1 : Sum  OutDataTypeStr=fixdt(0, ceil(log2(2*maxRho)), 0)  RndMeth=Round
  Compare To Constant1 : simulink/Logic and Bit Operations/Compare To Constant  relop===  const=width/2-1  OutDataTypeStr=boolean
  Constant : Constant  Value=maxRho  OutDataTypeStr=fixdt(0, ceil(log2(maxRho + 1)), 0);  SampleTime=-1
  Data Type Conversion : DataTypeConversion  OutDataTypeStr=uint8
  Hough Kernel : Subsystem
  Look Ahead Hough : Subsystem
  vEdge : Outport  VectorParamsAs1DForOutWhenUnconnected=off
  Rho : Outport  Port=2  VectorParamsAs1DForOutWhenUnconnected=off
  wires:
  Add1/1 -> Rho/1
  Compare To Constant1/1 -> Look Ahead Hough/2(eol)
  Constant/1 -> Add1/2
  Data Type Conversion/1 -> Hough Kernel/3(Index)
  Hough Kernel/1(Rho) -> Add1/1
  Look Ahead Hough/1(ysin) -> Hough Kernel/2(Y)
  Edge/1 -> vEdge/1
  X/1 -> Compare To Constant1/1, Hough Kernel/1(X)
  Y/1 -> Look Ahead Hough/1(Y)
  Index/1 -> Data Type Conversion/1
